simulink model "self_balancing_robot"  (R2017a)
settings: Solver=VariableStepAuto  StartTime=0.0  StopTime=10  RelTol=1e-3
values from neighbouring files (symbols this model uses):
  b = 0.1    [setup.m]
  g = 9.8    [setup.m]
  I = 0.006    [setup.m]
  Kd = 5    [setup.m]
  Ki = 20    [setup.m]
  Kp = 7    [setup.m]
  l = 0.2    [setup.m]
  m = 0.2    [setup.m]
  M = 0.3    [setup.m]
  q = (m+M)*(I+m*l^2)-(m*l)^2    (= 0.0054)    [setup.m]
undefined symbols (not defined in the file or in its folder): A, B, C, D
libraries: simulink x1
settings Model: Creator=Horia  LastModifiedBy=Horia

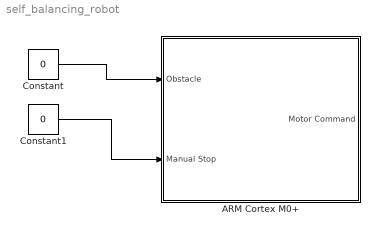
== system self_balancing_robot ==
  ARM Cortex M0+ : Subsystem
  Constant : Constant  Value=0
  Constant1 : Constant  Value=0
  wires:
  Constant/1 -> ARM Cortex M0+/1(Obstacle)
  Constant1/1 -> ARM Cortex M0+/2(Manual Stop)

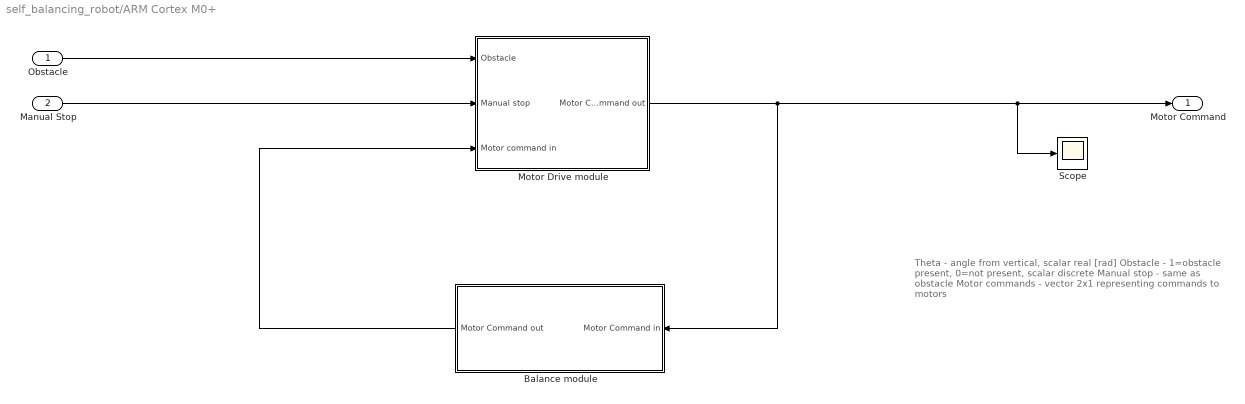
== system self_balancing_robot/ARM Cortex M0+ ==
  note: Theta - angle from vertical, scalar real [rad]
      | Obstacle - 1=obstacle present, 0=not present, scalar discrete
      | Manual stop - same as obstacle
      | Motor commands - vector 2x1 representing commands to motors
  Obstacle : Inport
  Manual Stop : Inport  Port=2
  Balance module : Subsystem
  Motor Drive module : Subsystem
  Scope : Scope
  Motor Command : Outport
  wires:
  Manual Stop/1 -> Motor Drive module/2(Manual stop)
  Obstacle/1 -> Motor Drive module/1(Obstacle)
  Balance module/1(Motor Command out) -> Motor Drive module/3(Motor command in)
  Motor Drive module/1(Motor Command out) -> Balance module/1(Motor Command in), Scope/1, Motor Command/1

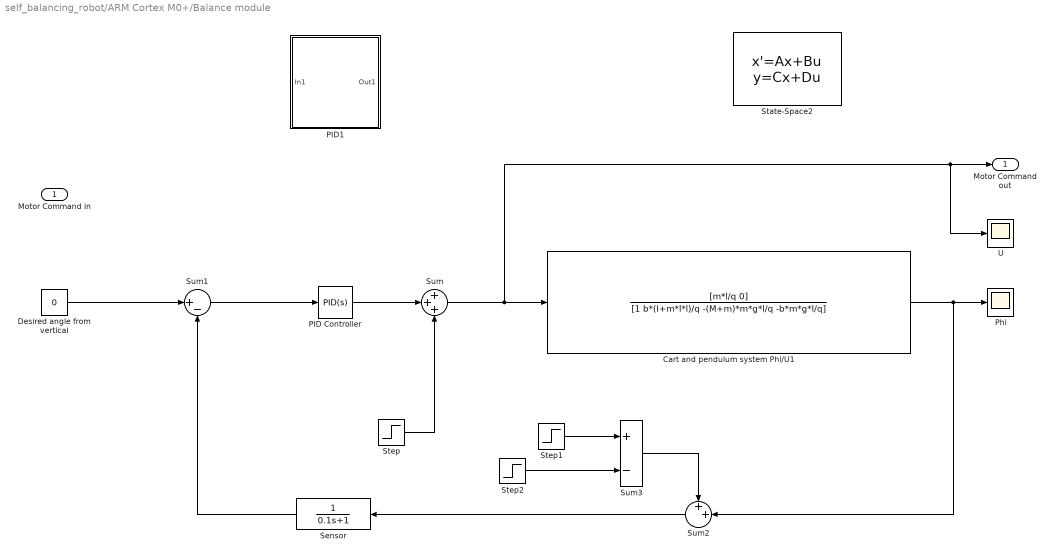
== system self_balancing_robot/ARM Cortex M0+/Balance module ==
  Motor Command in : Inport
  Cart and pendulum system Phi/U1 : TransferFcn  Numerator=[m*l/q 0]  Denominator=[1 b*(I+m*l*l)/q -(M+m)*m*g*l/q -b*m*g*l/q]
  Desired angle from vertical : Constant  Value=0
  PID Controller : simulink/Continuous/PID Controller  Controller=PID  TimeDomain=Continuous-time  SampleTime=-1  IntegratorMethod=Forward Euler  FilterMethod=Forward Euler  Form=Parallel  UseFilter=on  ControllerParametersSource=internal  P=69.6609184248737  I=20.2207036745879  D=18.855379703885  N=4147.68884072985  InitialConditionSource=internal  InitialConditionForIntegrator=0  InitialConditionForFilter=0  ExternalReset=none  LimitOutput=off  UpperSaturationLimit=inf  LowerSaturationLimit=-inf  LinearizeAsGain=on  AntiWindupMode=none  Kb=1  TrackingMode=off  Kt=1  PParamMin=[]  PParamMax=[]  IParamMin=[]  IParamMax=[]  DParamMin=[]  DParamMax=[]  NParamMin=[]  NParamMax=[]  KbParamMin=[]  KbParamMax=[]  KtParamMin=[]  KtParamMax=[]  POutMin=[]  POutMax=[]  IOutMin=[]  IOutMax=[]  DOutMin=[]  DOutMax=[]  NOutMin=[]  NOutMax=[]  KbOutMin=[]  KbOutMax=[]  KtOutMin=[]  KtOutMax=[]  IntegratorOutMin=[]  IntegratorOutMax=[]  FilterOutMin=[]  FilterOutMax=[]  SumOutMin=[]  SumOutMax=[]  SumI1OutMin=[]  SumI1OutMax=[]  SumI2OutMin=[]  SumI2OutMax=[]  SumI3OutMin=[]  SumI3OutMax=[]  SumDOutMin=[]  SumDOutMax=[]  SaturationOutMin=[]  SaturationOutMax=[]  IntegratorContinuousStateAttributes=''  IntegratorStateMustResolveToSignalObject=off  IntegratorRTWStateStorageClass=Auto  FilterContinuousStateAttributes=''  FilterStateMustResolveToSignalObject=off  FilterRTWStateStorageClass=Auto  DifferentiatorICPrevScaledInput=0  DifferentiatorOutMin=[]  DifferentiatorOutMax=[]  InitialConditionSetting=State (most efficient)
  PID1 : Subsystem
  Phi : Scope
  Sensor : TransferFcn  Denominator=[0.1 1]
  State-Space2 : StateSpace  A=A  B=B  C=C  D=D  X0=[0 0.4 0]
  Step : Step  After=0  SampleTime=0
  Step1 : Step  After=0.1  SampleTime=0
  Step2 : Step  Time=1.1  After=0.1  SampleTime=0
  Sum : Sum  Inputs=+++
  Sum1 : Sum  Inputs=|+-
  Sum2 : Sum  Inputs=++|
  Sum3 : Sum  Inputs=+-
  U : Scope
  Motor Command out : Outport
  wires:
  Desired angle from vertical/1 -> Sum1/1
  Sum1/1 -> PID Controller/1
  Sensor/1 -> Sum1/2
  Cart and pendulum system Phi/U1/1 -> Sum2/2, Phi/1
  Sum/1 -> U/1, Motor Command out/1, Cart and pendulum system Phi/U1/1
  Sum2/1 -> Sensor/1
  Sum3/1 -> Sum2/1
  Step1/1 -> Sum3/1
  Step2/1 -> Sum3/2
  PID Controller/1 -> Sum/2
  Step/1 -> Sum/3

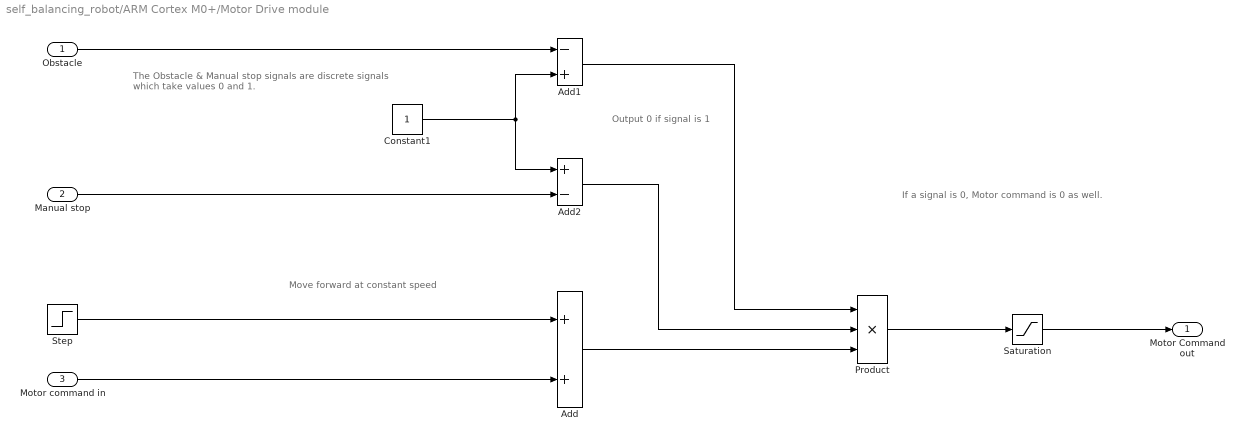
== system self_balancing_robot/ARM Cortex M0+/Motor Drive module ==
  note: Output 0 if signal is 1
  note: Move forward at constant speed
  note: If a signal is 0, Motor command is 0 as well.
  note: The Obstacle & Manual stop signals are discrete signals
      | which take values 0 and 1.
  Obstacle : Inport
  Manual stop : Inport  Port=2
  Motor command in : Inport  Port=3
  Add : Sum
  Add1 : Sum  Inputs=-+
  Add2 : Sum  Inputs=+-
  Constant1 : Constant
  Product : Product  Inputs=3
  Saturation : Saturate  UpperLimit=+4  LowerLimit=-4
  Step : Step  SampleTime=0
  Motor Command out : Outport
  wires:
  Product/1 -> Saturation/1
  Add/1 -> Product/3
  Step/1 -> Add/1
  Add1/1 -> Product/1
  Obstacle/1 -> Add1/1
  Constant1/1 -> Add2/1, Add1/2
  Manual stop/1 -> Add2/2
  Add2/1 -> Product/2
  Motor command in/1 -> Add/2
  Saturation/1 -> Motor Command out/1

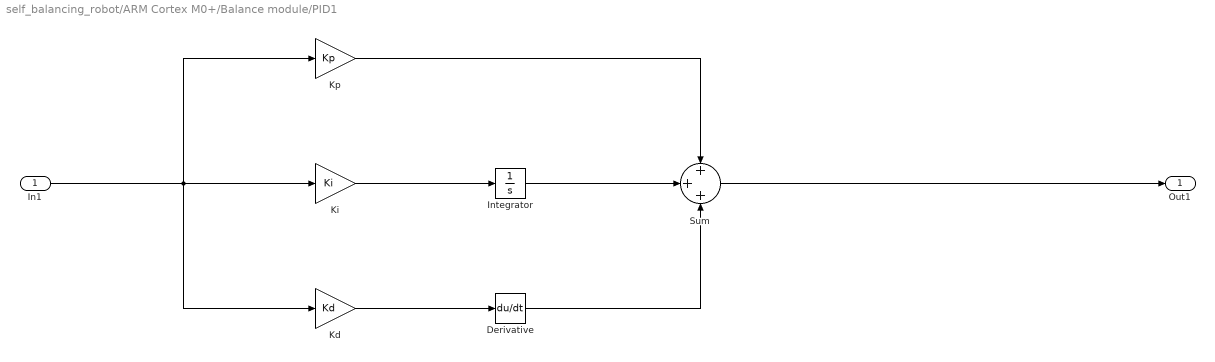
== system self_balancing_robot/ARM Cortex M0+/Balance module/PID1 ==
  In1 : Inport
  Derivative : Derivative
  Integrator : Integrator
  Kd : Gain  Gain=Kd
  Ki : Gain  Gain=Ki
  Kp : Gain  Gain=Kp
  Sum : Sum  Inputs=+++
  Out1 : Outport
  wires:
  Derivative/1 -> Sum/3
  Kd/1 -> Derivative/1
  Integrator/1 -> Sum/2
  Ki/1 -> Integrator/1
  In1/1 -> Kp/1, Ki/1, Kd/1
  Kp/1 -> Sum/1
  Sum/1 -> Out1/1
